simulink library "eng_simple_transient_std"  (Simulink 8.7)
settings: Solver=ode45  StartTime=0.0  StopTime=10.0  RelTol=1e-3
undefined symbols (not defined in the file): DiscIntNeverNeededParam, sMP
libraries: simulink x17
(part 1 of 3)
settings Model: Creator=rafrey5  LastModifiedBy=gerhajo

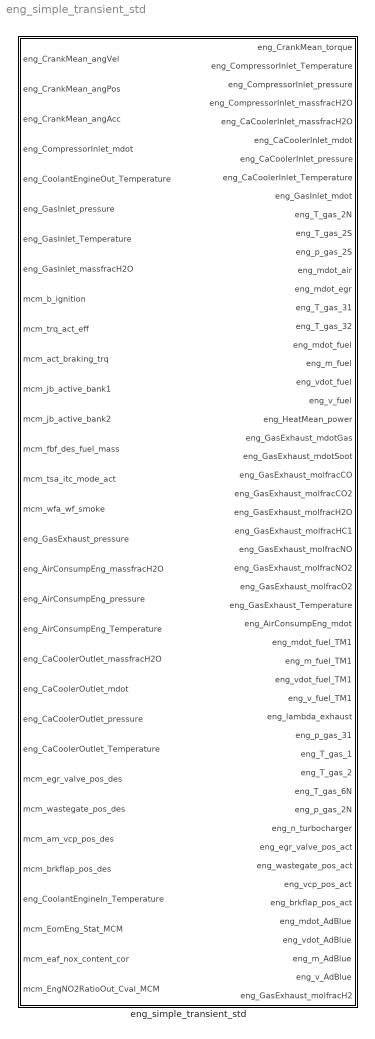
== system eng_simple_transient_std ==
  eng_simple_transient_std : Subsystem  TreatAsAtomicUnit=on  SystemSampleTime=0.01  mask{Airpath_EGRcooler_x_EGR_flow=sMP.phys.eng.Airpath_EGRcooler_x_EGR_flow, Airpath_EGRcooler_y_delta_Temp=sMP.phys.eng.Airpath_EGRcooler_y_delta_Temp, Airpath_EGRcooler_z_efficiency=sMP.phys.eng.Airpath_EGRcooler_z_efficiency, Airpath_Pdrop_aftTurb_coeff=sMP.phys.eng.Airpath_Pdrop_aftTurb_coeff, Airpath_Pdrop_aircooler_coeff=sMP.phys.eng.Airpath_Pdrop_aircooler_coeff, Airpath_Pdrop_aircooler_coeffBr_a1=sMP.phys.eng.Airpath_Pdrop_aircooler_coeffBr_a1, Airpath_Pdrop_aircooler_coeffBr_a2=sMP.phys.eng.Airpath_Pdrop_aircooler_coeffBr_a2, Airpath_Pdrop_bfrComp_coeff=sMP.phys.eng.Airpath_Pdrop_bfrComp_coeff, Airpath_Tairbox_EGR_coeff=sMP.phys.eng.Airpath_Tairbox_EGR_coeff, Airpath_aircooler_x_ML_kgh=sMP.phys.eng.Airpath_aircooler_x_ML_kgh, Airpath_aircooler_y_delta_Temp=sMP.phys.eng.Airpath_aircooler_y_delta_Temp, Airpath_aircooler_z_efficiency=sMP.phys.eng.Airpath_aircooler_z_efficiency, Airpath_compressor_x_massFlow_kgh=sMP.phys.eng.Airpath_compressor_x_massFlow_kgh, Airpath_compressor_y_PressRatio=sMP.phys.eng.Airpath_compressor_y_PressRatio, Airpath_compressor_z_Efficiency=sMP.phys.eng.Airpath_compressor_z_Efficiency, Airpath_intakeflow_x_NMOTW_rpm=sMP.phys.eng.Airpath_intakeflow_x_NMOTW_rpm, Airpath_intakeflow_y_P2S_mbar=sMP.phys.eng.Airpath_intakeflow_y_P2S_mbar, Airpath_intakeflow_z_VolEff=sMP.phys.eng.Airpath_intakeflow_z_VolEff, Airpath_turbine_x_PressRatio=sMP.phys.eng.Airpath_turbine_x_PressRatio, Airpath_turbine_y_Efficiency=sMP.phys.eng.Airpath_turbine_y_Efficiency, ECU_torque_x_NMOT_rpm=sMP.phys.eng.ECU_torque_x_NMOT_rpm, ECU_torque_y_FrictionLine_MISTEE_Nm=sMP.phys.eng.ECU_torque_y_FrictionLine_MISTEE_Nm, ECU_torque_y_FullLoad_MISTEE_Nm=sMP.phys.eng.ECU_torque_y_FullLoad_MISTEE_Nm, Eng_characteristics_AdBlue_density=sMP.phys.eng.Eng_characteristics_AdBlue_density, Eng_characteristics_Fuel_density=sMP.phys.eng.Eng_characteristics_Fuel_density, Eng_characteristics_Mfuel_available=sMP.phys.eng.Eng_characteristics_Mfuel_available, Eng_characteristics_Mfuel_with_MCM=sMP.phys.eng.Eng_characteristics_Mfuel_with_MCM, Eng_characteristics_Stoech_coeff=sMP.phys.eng.Eng_characteristics_Stoech_coeff, Eng_characteristics_V_cylinder=sMP.phys.eng.Eng_characteristics_V_cylinder, Eng_characteristics_assymTurbine=sMP.phys.eng.Eng_characteristics_assymTurbine, Eng_characteristics_n_cylinder=sMP.phys.eng.Eng_characteristics_n_cylinder, Eng_characteristics_use_mcm_NOx=sMP.phys.eng.Eng_characteristics_use_mcm_NOx, Eng_initialisation_eng_started=sMP.phys.eng.Eng_initialisation_eng_started, Eng_starter_fuelInj_minEngSpd=sMP.phys.eng.Eng_starter_fuelInj_minEngSpd, Eng_starter_fuel_penalty_kg=sMP.phys.eng.Eng_starter_fuel_penalty_kg, Eng_starter_time_constant=sMP.phys.eng.Eng_starter_time_constant, Eng_starter_torque_Nm=sMP.phys.eng.Eng_starter_torque_Nm, Fiter_calibration_brmode_x_NMOT_rpm=sMP.phys.eng.Fiter_calibration_brmode_x_NMOT_rpm, Fiter_calibration_brmode_y_tc_P2S=sMP.phys.eng.Fiter_calibration_brmode_y_tc_P2S, Fiter_calibration_brmode_y_tc_P31=sMP.phys.eng.Fiter_calibration_brmode_y_tc_P31, Fiter_calibration_brmode_y_tc_P32=sMP.phys.eng.Fiter_calibration_brmode_y_tc_P32, Fiter_calibration_brmode_y_tc_T31=sMP.phys.eng.Fiter_calibration_brmode_y_tc_T31, Fiter_calibration_brmode_y_tc_T32=sMP.phys.eng.Fiter_calibration_brmode_y_tc_T32, Fiter_calibration_dt=sMP.phys.eng.Fiter_calibration_dt, Fiter_calibration_fmode_x_NMOT_rpm=sMP.phys.eng.Fiter_calibration_fmode_x_NMOT_rpm, Fiter_calibration_fmode_y_ec_EGRTAT=sMP.phys.eng.Fiter_calibration_fmode_y_ec_EGRTAT, Fiter_calibration_fmode_y_tc_EGRTAT=sMP.phys.eng.Fiter_calibration_fmode_y_tc_EGRTAT, Fiter_calibration_fmode_y_tc_P2S_dc=sMP.phys.eng.Fiter_calibration_fmode_y_tc_P2S_dc, Fiter_calibration_fmode_y_tc_P2S_ic=sMP.phys.eng.Fiter_calibration_fmode_y_tc_P2S_ic, Fiter_calibration_fmode_y_tc_P31_dc=sMP.phys.eng.Fiter_calibration_fmode_y_tc_P31_dc, Fiter_calibration_fmode_y_tc_P31_ic=sMP.phys.eng.Fiter_calibration_fmode_y_tc_P31_ic, Fiter_calibration_fmode_y_tc_P32_dc=sMP.phys.eng.Fiter_calibration_fmode_y_tc_P32_dc, Fiter_calibration_fmode_y_tc_P32_ic=sMP.phys.eng.Fiter_calibration_fmode_y_tc_P32_ic, Fiter_calibration_fmode_y_tc_T2N=sMP.phys.eng.Fiter_calibration_fmode_y_tc_T2N, Fiter_calibration_fmode_y_tc_T2V=sMP.phys.eng.Fiter_calibration_fmode_y_tc_T2V, Fiter_calibration_fmode_y_tc_T31_dc=sMP.phys.eng.Fiter_calibration_fmode_y_tc_T31_dc, Fiter_calibration_fmode_y_tc_T31_ic=sMP.phys.eng.Fiter_calibration_fmode_y_tc_T31_ic, Fiter_calibration_fmode_y_tc_T32_dc=sMP.phys.eng.Fiter_calibration_fmode_y_tc_T32_dc, Fiter_calibration_fmode_y_tc_T32_ic=sMP.phys.eng.Fiter_calibration_fmode_y_tc_T32_ic, Setpoint_brakingMode1_x_NMOTW_rpm=sMP.phys.eng.Setpoint_brakingMode1_x_NMOTW_rpm, Setpoint_brakingMode1_y_alphaTorque=sMP.phys.eng.Setpoint_brakingMode1_y_alphaTorque, Setpoint_brakingMode1_z_P2S_mbar=sMP.phys.eng.Setpoint_brakingMode1_z_P2S_mbar, Setpoint_brakingMode1_z_P31_mbar=sMP.phys.eng.Setpoint_brakingMode1_z_P31_mbar, Setpoint_brakingMode1_z_T31_degC=sMP.phys.eng.Setpoint_brakingMode1_z_T31_degC, Setpoint_brakingMode1_z_Torque_Nm=sMP.phys.eng.Setpoint_brakingMode1_z_Torque_Nm, Setpoint_brakingMode2_x_NMOTW_rpm=sMP.phys.eng.Setpoint_brakingMode2_x_NMOTW_rpm, Setpoint_brakingMode2_y_alphaTorque=sMP.phys.eng.Setpoint_brakingMode2_y_alphaTorque, Setpoint_brakingMode2_z_P2S_mbar=sMP.phys.eng.Setpoint_brakingMode2_z_P2S_mbar, Setpoint_brakingMode2_z_P32_mbar=sMP.phys.eng.Setpoint_brakingMode2_z_P32_mbar, Setpoint_brakingMode2_z_T32_degC=sMP.phys.eng.Setpoint_brakingMode2_z_T32_degC, Setpoint_brakingMode2_z_Torque_Nm=sMP.phys.eng.Setpoint_brakingMode2_z_Torque_Nm, Setpoint_brakingMode3_x_NMOTW_rpm=sMP.phys.eng.Setpoint_brakingMode3_x_NMOTW_rpm, Setpoint_brakingMode3_y_alphaTorque=sMP.phys.eng.Setpoint_brakingMode3_y_alphaTorque, Setpoint_brakingMode3_z_EGRTAT=sMP.phys.eng.Setpoint_brakingMode3_z_EGRTAT, Setpoint_brakingMode3_z_P2S_mbar=sMP.phys.eng.Setpoint_brakingMode3_z_P2S_mbar, Setpoint_brakingMode3_z_P31_mbar=sMP.phys.eng.Setpoint_brakingMode3_z_P31_mbar, Setpoint_brakingMode3_z_P32_mbar=sMP.phys.eng.Setpoint_brakingMode3_z_P32_mbar, Setpoint_brakingMode3_z_T31_degC=sMP.phys.eng.Setpoint_brakingMode3_z_T31_degC, Setpoint_brakingMode3_z_T32_degC=sMP.phys.eng.Setpoint_brakingMode3_z_T32_degC, Setpoint_brakingMode3_z_Torque_Nm=sMP.phys.eng.Setpoint_brakingMode3_z_Torque_Nm, Setpoint_fuelledMode_x_NMOTW_rpm=sMP.phys.eng.Setpoint_fuelledMode_x_NMOTW_rpm, Setpoint_fuelledMode_y_alphaTorque=sMP.phys.eng.Setpoint_fuelledMode_y_alphaTorque, Setpoint_fuelledMode_z_CO_ppm=sMP.phys.eng.Setpoint_fuelledMode_z_CO_ppm, Setpoint_fuelledMode_z_dMFueldT2N=sMP.phys.eng.Setpoint_fuelledMode_z_dMFueldT2N, Setpoint_fuelledMode_z_dMFueldTWE=sMP.phys.eng.Setpoint_fuelledMode_z_dMFueldTWE, Setpoint_fuelledMode_z_EGRTAT=sMP.phys.eng.Setpoint_fuelledMode_z_EGRTAT, Setpoint_fuelledMode_z_HC_ppm=sMP.phys.eng.Setpoint_fuelledMode_z_HC_ppm, Setpoint_fuelledMode_z_MAdBlue_kgh=sMP.phys.eng.Setpoint_fuelledMode_z_MAdBlue_kgh, Setpoint_fuelledMode_z_Mfuel_mgstr=sMP.phys.eng.Setpoint_fuelledMode_z_Mfuel_mgstr, Setpoint_fuelledMode_z_Mfuel_TM1_mgstr=sMP.phys.eng.Setpoint_fuelledMode_z_Mfuel_TM1_mgstr, Setpoint_fuelledMode_z_Mfuel_smoke_factor=sMP.phys.eng.Setpoint_fuelledMode_z_Mfuel_smoke_factor, Setpoint_fuelledMode_z_NO_ppm=sMP.phys.eng.Setpoint_fuelledMode_z_NO_ppm, Setpoint_fuelledMode_z_NOx_ppm=sMP.phys.eng.Setpoint_fuelledMode_z_NOx_ppm, Setpoint_fuelledMode_z_P2S_mbar=sMP.phys.eng.Setpoint_fuelledMode_z_P2S_mbar, Setpoint_fuelledMode_z_P31_mbar=sMP.phys.eng.Setpoint_fuelledMode_z_P31_mbar, Setpoint_fuelledMode_z_P32_mbar=sMP.phys.eng.Setpoint_fuelledMode_z_P32_mbar, Setpoint_fuelledMode_z_T2N_degC=sMP.phys.eng.Setpoint_fuelledMode_z_T2N_degC, Setpoint_fuelledMode_z_T31_degC=sMP.phys.eng.Setpoint_fuelledMode_z_T31_degC, Setpoint_fuelledMode_z_T32_degC=sMP.phys.eng.Setpoint_fuelledMode_z_T32_degC, Setpoint_fuelledMode_z_TWE_degC=sMP.phys.eng.Setpoint_fuelledMode_z_TWE_degC, Setpoint_fuelledMode_z_Torque_Nm=sMP.phys.eng.Setpoint_fuelledMode_z_Torque_Nm, Thermal_heatRelease_negTorque_factor=sMP.phys.eng.Thermal_heatRelease_negTorque_factor, Thermal_heatRelease_x_NMOT_rpm=sMP.phys.eng.Thermal_heatRelease_x_NMOT_rpm, Thermal_heatRelease_y_Torque_Nm=sMP.phys.eng.Thermal_heatRelease_y_Torque_Nm, Thermal_heatRelease_z_heat_kW=sMP.phys.eng.Thermal_heatRelease_z_heat_kW, egr_smoke_lim_x_NMOT_rpm=sMP.phys.eng.egr_smoke_lim_x_NMOT_rpm, egr_smoke_lim_y_Mfuel_mgstr=sMP.phys.eng.egr_smoke_lim_y_Mfuel_mgstr, egr_smoke_lim_z_desAir_kgh=sMP.phys.eng.egr_smoke_lim_z_desAir_kgh, egr_smoke_lim_z_minAFR=sMP.phys.eng.egr_smoke_lim_z_minAFR, tc_speed_calc_3m=sMP.phys.eng.tc_speed_calc_3m, tc_speed_calc_x_p_intake=sMP.phys.eng.tc_speed_calc_x_p_intake, tc_speed_calc_y_eng_speed=sMP.phys.eng.tc_speed_calc_y_eng_speed}
      mask init:
      | 0.01;
      mask Display: disp(['Fast engine model' char(10) 'Release date :' char(10) '2021 / 07 / 21'])

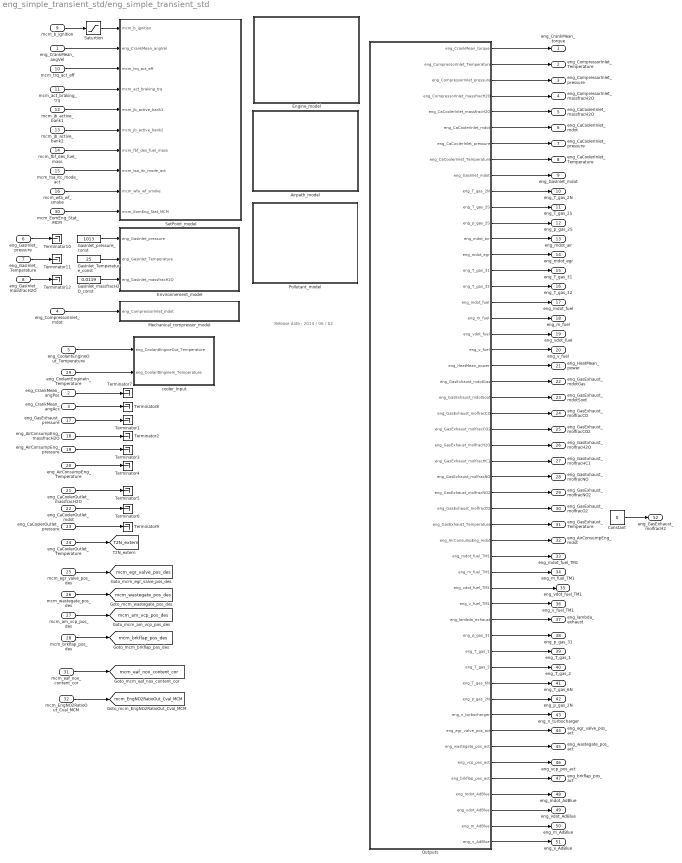
== system eng_simple_transient_std/eng_simple_transient_std ==
  note: Release date :
      | 2014 / 06 / 02
  eng_CrankMean_angVel : Inport
  eng_CrankMean_angPos : Inport  Port=2
  eng_CrankMean_angAcc : Inport  Port=3
  eng_CompressorInlet_mdot : Inport  Port=4
  eng_CoolantEngineOut_Temperature : Inport  Port=5
  eng_GasInlet_pressure : Inport  Port=6
  eng_GasInlet_Temperature : Inport  Port=7
  eng_GasInlet_massfracH2O : Inport  Port=8
  mcm_b_ignition : Inport  Port=9
  mcm_trq_act_eff : Inport  Port=10
  mcm_act_braking_trq : Inport  Port=11
  mcm_jb_active_bank1 : Inport  Port=12
  mcm_jb_active_bank2 : Inport  Port=13
  mcm_fbf_des_fuel_mass : Inport  Port=14
  mcm_tsa_itc_mode_act : Inport  Port=15
  mcm_wfa_wf_smoke : Inport  Port=16
  eng_GasExhaust_pressure : Inport  Port=17
  eng_AirConsumpEng_massfracH2O : Inport  Port=18
  eng_AirConsumpEng_pressure : Inport  Port=19
  eng_AirConsumpEng_Temperature : Inport  Port=20
  eng_CaCoolerOutlet_massfracH2O : Inport  Port=21
  eng_CaCoolerOutlet_mdot : Inport  Port=22
  eng_CaCoolerOutlet_pressure : Inport  Port=23
  eng_CaCoolerOutlet_Temperature : Inport  Port=24
  mcm_egr_valve_pos_des : Inport  Port=25
  mcm_wastegate_pos_des : Inport  Port=26
  mcm_am_vcp_pos_des : Inport  Port=27
  mcm_brkflap_pos_des : Inport  Port=28
  eng_CoolantEngineIn_Temperature : Inport  Port=29
  mcm_EomEng_Stat_MCM : Inport  Port=30
  mcm_eaf_nox_content_cor : Inport  Port=31
  mcm_EngNO2RatioOut_Cval_MCM : Inport  Port=32
  Airpath_model : Subsystem
  Constant : Constant  Value=0
  Engine_model : Subsystem
  Environnement_model : Subsystem
  GasInlet_Temperature_const : Constant  Value=25
  GasInlet_massfracH2O_const : Constant  Value=0.0119
  GasInlet_pressure_const : Constant  Value=1013
  Mechanical_compressor_model : Subsystem
  Outputs : Subsystem
  Pollutant_model : Subsystem
  Saturtion : Saturate  UpperLimit=1  LowerLimit=1
  SetPoint_model : Subsystem
  Terminator{1..12} (12 alike) : Terminator
  cooler_Input : Subsystem
  eng_CrankMean_torque : Outport
  eng_CompressorInlet_Temperature : Outport  Port=2
  eng_CompressorInlet_pressure : Outport  Port=3
  eng_CompressorInlet_massfracH2O : Outport  Port=4
  eng_CaCoolerInlet_massfracH2O : Outport  Port=5
  eng_CaCoolerInlet_mdot : Outport  Port=6
  eng_CaCoolerInlet_pressure : Outport  Port=7
  eng_CaCoolerInlet_Temperature : Outport  Port=8
  eng_GasInlet_mdot : Outport  Port=9
  eng_T_gas_2N : Outport  Port=10
  eng_T_gas_2S : Outport  Port=11
  eng_p_gas_2S : Outport  Port=12
  eng_mdot_air : Outport  Port=13
  eng_mdot_egr : Outport  Port=14
  eng_T_gas_31 : Outport  Port=15
  eng_T_gas_32 : Outport  Port=16
  eng_mdot_fuel : Outport  Port=17
  eng_m_fuel : Outport  Port=18
  eng_vdot_fuel : Outport  Port=19
  eng_v_fuel : Outport  Port=20
  eng_HeatMean_power : Outport  Port=21
  eng_GasExhaust_mdotGas : Outport  Port=22
  eng_GasExhaust_mdotSoot : Outport  Port=23
  eng_GasExhaust_molfracCO : Outport  Port=24
  eng_GasExhaust_molfracCO2 : Outport  Port=25
  eng_GasExhaust_molfracH2O : Outport  Port=26
  eng_GasExhaust_molfracHC1 : Outport  Port=27
  eng_GasExhaust_molfracNO : Outport  Port=28
  eng_GasExhaust_molfracNO2 : Outport  Port=29
  eng_GasExhaust_molfracO2 : Outport  Port=30
  eng_GasExhaust_Temperature : Outport  Port=31
  eng_AirConsumpEng_mdot : Outport  Port=32
  eng_mdot_fuel_TM1 : Outport  Port=33
  eng_m_fuel_TM1 : Outport  Port=34
  eng_vdot_fuel_TM1 : Outport  Port=35
  eng_v_fuel_TM1 : Outport  Port=36
  eng_lambda_exhaust : Outport  Port=37
  eng_p_gas_31 : Outport  Port=38
  eng_T_gas_1 : Outport  Port=39
  eng_T_gas_2 : Outport  Port=40
  eng_T_gas_6N : Outport  Port=41
  eng_p_gas_2N : Outport  Port=42
  eng_n_turbocharger : Outport  Port=43
  eng_egr_valve_pos_act : Outport  Port=44
  eng_wastegate_pos_act : Outport  Port=45
  eng_vcp_pos_act : Outport  Port=46
  eng_brkflap_pos_act : Outport  Port=47
  eng_mdot_AdBlue : Outport  Port=48
  eng_vdot_AdBlue : Outport  Port=49
  eng_m_AdBlue : Outport  Port=50
  eng_v_AdBlue : Outport  Port=51
  eng_GasExhaust_molfracH2 : Outport  Port=52
  tag scope: T2N_extern=global, mcm_EngNO2RatioOut_Cval_MCM=global, mcm_am_vcp_pos_des=global, mcm_brkflap_pos_des=global, mcm_eaf_nox_content_cor=global, mcm_egr_valve_pos_des=global, mcm_wastegate_pos_des=global
  wires:
  eng_CompressorInlet_mdot/1 -> Mechanical_compressor_model/1(eng_CompressorInlet_mdot)
  eng_CrankMean_angVel/1 -> SetPoint_model/2(eng_CrankMean_angVel)
  eng_CrankMean_angAcc/1 -> Terminator8/1
  eng_CrankMean_angPos/1 -> Terminator7/1
  eng_CoolantEngineOut_Temperature/1 -> cooler_Input/1(eng_CoolantEngineOut_Temperature)
  mcm_fbf_des_fuel_mass/1 -> SetPoint_model/7(mcm_fbf_des_fuel_mass)
  mcm_jb_active_bank2/1 -> SetPoint_model/6(mcm_jb_active_bank2)
  mcm_jb_active_bank1/1 -> SetPoint_model/5(mcm_jb_active_bank1)
  mcm_act_braking_trq/1 -> SetPoint_model/4(mcm_act_braking_trq)
  mcm_trq_act_eff/1 -> SetPoint_model/3(mcm_trq_act_eff)
  mcm_b_ignition/1 -> Saturtion/1
  eng_GasExhaust_pressure/1 -> Terminator1/1
  eng_AirConsumpEng_massfracH2O/1 -> Terminator2/1
  eng_AirConsumpEng_pressure/1 -> Terminator3/1
  eng_AirConsumpEng_Temperature/1 -> Terminator4/1
  Saturtion/1 -> SetPoint_model/1(mcm_b_ignition)
  mcm_tsa_itc_mode_act/1 -> SetPoint_model/8(mcm_tsa_itc_mode_act)
  mcm_wfa_wf_smoke/1 -> SetPoint_model/9(mcm_wfa_wf_smoke)
  Outputs/1(eng_CrankMean_torque) -> eng_CrankMean_torque/1
  Outputs/2(eng_CompressorInlet_Temperature) -> eng_CompressorInlet_Temperature/1
  Outputs/3(eng_CompressorInlet_pressure) -> eng_CompressorInlet_pressure/1
  Outputs/4(eng_CompressorInlet_massfracH2O) -> eng_CompressorInlet_massfracH2O/1
  Outputs/5(eng_CaCoolerInlet_massfracH2O) -> eng_CaCoolerInlet_massfracH2O/1
  Outputs/6(eng_CaCoolerInlet_mdot) -> eng_CaCoolerInlet_mdot/1
  Outputs/7(eng_CaCoolerInlet_pressure) -> eng_CaCoolerInlet_pressure/1
  Outputs/8(eng_CaCoolerInlet_Temperature) -> eng_CaCoolerInlet_Temperature/1
  Outputs/9(eng_GasInlet_mdot) -> eng_GasInlet_mdot/1
  Outputs/10(eng_T_gas_2N) -> eng_T_gas_2N/1
  Outputs/11(eng_T_gas_2S) -> eng_T_gas_2S/1
  Outputs/12(eng_p_gas_2S) -> eng_p_gas_2S/1
  Outputs/13(eng_mdot_air) -> eng_mdot_air/1
  Outputs/14(eng_mdot_egr) -> eng_mdot_egr/1
  Outputs/15(eng_T_gas_31) -> eng_T_gas_31/1
  Outputs/16(eng_T_gas_32) -> eng_T_gas_32/1
  Outputs/17(eng_mdot_fuel) -> eng_mdot_fuel/1
  Outputs/18(eng_m_fuel) -> eng_m_fuel/1
  Outputs/19(eng_vdot_fuel) -> eng_vdot_fuel/1
  Outputs/20(eng_v_fuel) -> eng_v_fuel/1
  Outputs/21(eng_HeatMean_power) -> eng_HeatMean_power/1
  Outputs/22(eng_GasExhaust_mdotGas) -> eng_GasExhaust_mdotGas/1
  Outputs/23(eng_GasExhaust_mdotSoot) -> eng_GasExhaust_mdotSoot/1
  Outputs/24(eng_GasExhaust_molfracCO) -> eng_GasExhaust_molfracCO/1
  Outputs/25(eng_GasExhaust_molfracCO2) -> eng_GasExhaust_molfracCO2/1
  Outputs/26(eng_GasExhaust_molfracH2O) -> eng_GasExhaust_molfracH2O/1
  Outputs/27(eng_GasExhaust_molfracHC1) -> eng_GasExhaust_molfracHC1/1
  Outputs/28(eng_GasExhaust_molfracNO) -> eng_GasExhaust_molfracNO/1
  Outputs/29(eng_GasExhaust_molfracNO2) -> eng_GasExhaust_molfracNO2/1
  Outputs/30(eng_GasExhaust_molfracO2) -> eng_GasExhaust_molfracO2/1
  Outputs/31(eng_GasExhaust_Temperature) -> eng_GasExhaust_Temperature/1
  Outputs/32(eng_AirConsumpEng_mdot) -> eng_AirConsumpEng_mdot/1
  eng_CaCoolerOutlet_massfracH2O/1 -> Terminator5/1
  eng_CaCoolerOutlet_mdot/1 -> Terminator6/1
  eng_CaCoolerOutlet_pressure/1 -> Terminator9/1
  eng_CaCoolerOutlet_Temperature/1 -> [T2N_extern]
  Outputs/33(eng_mdot_fuel_TM1) -> eng_mdot_fuel_TM1/1
  Outputs/34(eng_m_fuel_TM1) -> eng_m_fuel_TM1/1
  Outputs/35(eng_vdot_fuel_TM1) -> eng_vdot_fuel_TM1/1
  Outputs/36(eng_v_fuel_TM1) -> eng_v_fuel_TM1/1
  Outputs/37(eng_lambda_exhaust) -> eng_lambda_exhaust/1
  Outputs/38(eng_p_gas_31) -> eng_p_gas_31/1
  Outputs/39(eng_T_gas_1) -> eng_T_gas_1/1
  Outputs/40(eng_T_gas_2) -> eng_T_gas_2/1
  Outputs/41(eng_T_gas_6N) -> eng_T_gas_6N/1
  Outputs/42(eng_p_gas_2N) -> eng_p_gas_2N/1
  Outputs/43(eng_n_turbocharger) -> eng_n_turbocharger/1
  mcm_egr_valve_pos_des/1 -> [mcm_egr_valve_pos_des]
  mcm_wastegate_pos_des/1 -> [mcm_wastegate_pos_des]
  mcm_am_vcp_pos_des/1 -> [mcm_am_vcp_pos_des]
  mcm_brkflap_pos_des/1 -> [mcm_brkflap_pos_des]
  Outputs/44(eng_egr_valve_pos_act) -> eng_egr_valve_pos_act/1
  Outputs/45(eng_wastegate_pos_act) -> eng_wastegate_pos_act/1
  Outputs/46(eng_vcp_pos_act) -> eng_vcp_pos_act/1
  Outputs/47(eng_brkflap_pos_act) -> eng_brkflap_pos_act/1
  Outputs/48(eng_mdot_AdBlue) -> eng_mdot_AdBlue/1
  Outputs/49(eng_vdot_AdBlue) -> eng_vdot_AdBlue/1
  Outputs/50(eng_m_AdBlue) -> eng_m_AdBlue/1
  Outputs/51(eng_v_AdBlue) -> eng_v_AdBlue/1
  eng_CoolantEngineIn_Temperature/1 -> cooler_Input/2(eng_CoolantEngineIn_Temperature)
  mcm_EomEng_Stat_MCM/1 -> SetPoint_model/10(mcm_EomEng_Stat_MCM)
  mcm_eaf_nox_content_cor/1 -> [mcm_eaf_nox_content_cor]
  mcm_EngNO2RatioOut_Cval_MCM/1 -> [mcm_EngNO2RatioOut_Cval_MCM]
  Constant/1 -> eng_GasExhaust_molfracH2/1
  eng_GasInlet_massfracH2O/1 -> Terminator12/1
  eng_GasInlet_Temperature/1 -> Terminator11/1
  eng_GasInlet_pressure/1 -> Terminator10/1
  GasInlet_Temperature_const/1 -> Environnement_model/2(eng_GasInlet_Temperature)
  GasInlet_pressure_const/1 -> Environnement_model/1(eng_GasInlet_pressure)
  GasInlet_massfracH2O_const/1 -> Environnement_model/3(eng_GasInlet_massfracH2O)

== system eng_simple_transient_std/eng_simple_transient_std/Airpath_model ==
  After EGR cooler calculation : Subsystem
  After air cooler calculation : Subsystem
  After compressor calculation : Subsystem
  After turbine calculation : Subsystem
  Airbox calculation : Subsystem
  Before EGR cooler calculation : Subsystem
  Before compressor calculation : Subsystem
  Before turbine calculation : Subsystem
  Bus Creator4 : BusCreator  Inputs=22
  Intake flows calculation : Subsystem
  tag scope: Airpath=global
  wires:
  Before turbine calculation/4(T32_degC) -> Bus Creator4/16  "T32_degC"
  Before turbine calculation/3(P32_mbar) -> Bus Creator4/15  "P32_mbar"
  After EGR cooler calculation/2(T6N_degC) -> Bus Creator4/22  "T6N_degC"
  After EGR cooler calculation/1(P6N_mbar) -> Bus Creator4/21  "P6N_mbar"
  Before EGR cooler calculation/2(T6V_degC) -> Bus Creator4/20  "T6V_degC"
  Before EGR cooler calculation/1(P6V_mbar) -> Bus Creator4/19  "P6V_mbar"
  After turbine calculation/2(T4_degC) -> Bus Creator4/18  "T4_degC"
  After turbine calculation/1(P4_mbar) -> Bus Creator4/17  "P4_mbar"
  Before turbine calculation/2(T31_degC) -> Bus Creator4/14  "T31_degC"
  Before turbine calculation/1(P31_mbar) -> Bus Creator4/13  "P31_mbar"
  Airbox calculation/2(T2S_degC) -> Bus Creator4/12  "T2S_degC"
  Airbox calculation/1(P2S_mbar) -> Bus Creator4/11  "P2S_mbar"
  After air cooler calculation/2(T2N_degC) -> Bus Creator4/10  "T2N_degC"
  After air cooler calculation/1(P2N_mbar) -> Bus Creator4/9  "P2N_mbar"
  After compressor calculation/2(T2V_degC) -> Bus Creator4/8  "T2V_degC"
  After compressor calculation/1(P2V_mbar) -> Bus Creator4/7  "P2V_mbar"
  Before compressor calculation/3(T1_degC) -> Bus Creator4/6  "T1_degC"
  Before compressor calculation/2(P1_mbar) -> Bus Creator4/5  "P1_mbar"
  Before compressor calculation/1(massfracH2O) -> Bus Creator4/4  "massfracH2O"
  Intake flows calculation/3(EGRTAT) -> Bus Creator4/3  "EGRTAT"
  Intake flows calculation/2(EGR_flow_kgh) -> Bus Creator4/2  "EGRflow_kgh"
  Intake flows calculation/1(Air_mass_flow_kgh) -> Bus Creator4/1  "AirMassFlow_kgh"
  Bus Creator4/1 -> [Airpath]  "Airpath"

== system eng_simple_transient_std/eng_simple_transient_std/Engine_model ==
  AFR calculation : Subsystem
  AdBlue consumption : Subsystem
  Bus Creator4 : BusCreator  Inputs=17
  Fuel consumption calculation : Subsystem
  cooler_model : Subsystem
  tag scope: Engine=global
  wires:
  Bus Creator4/1 -> [Engine]  "Engine"
  Fuel consumption calculation/2(VFuel_Lh) -> Bus Creator4/4  "Vfuel_Lh"
  Fuel consumption calculation/4(VFuel_L) -> Bus Creator4/6  "Vfuel_L"
  Fuel consumption calculation/3(MFuel_kg) -> Bus Creator4/5  "Mfuel_kg"
  Fuel consumption calculation/1(MFuel_kgh) -> Bus Creator4/3  "Mfuel_kgh"
  [Mfuel_mgstr] -> Bus Creator4/2  "Mfuel_mgstr"
  [Torque_Nm_sp] -> Bus Creator4/1  "Torque_Nm"
  Fuel consumption calculation/5(MFuel_TM1_kgh) -> Bus Creator4/7  "Mfuel_TM1_kgh"
  Fuel consumption calculation/6(VFuel_TM1_Lh) -> Bus Creator4/8  "Vfuel_TM1_Lh"
  Fuel consumption calculation/7(MFuel_TM1_kg) -> Bus Creator4/9  "Mfuel_TM1_kg"
  Fuel consumption calculation/8(VFuel_TM1_L) -> Bus Creator4/10  "Vfuel_TM1_L"
  AFR calculation/1(AFR) -> Bus Creator4/11  "AFR"
  cooler_model/1(eng_HeatMean_power) -> Bus Creator4/12
  [EngSpeed] -> Bus Creator4/13  "EngSpeed_rpm"
  AdBlue consumption/1(MAdBlue_brk_kgh) -> Bus Creator4/14  "MAdBlue_kgh"
  AdBlue consumption/2(VAdBlue_Lh) -> Bus Creator4/15  "VAdBlue_Lh"
  AdBlue consumption/3(MAdBlue_kg) -> Bus Creator4/16  "MAdBlue_kg"
  AdBlue consumption/4(VAdBlue_L) -> Bus Creator4/17  "VAdBlue_L"

== system eng_simple_transient_std/eng_simple_transient_std/Environnement_model ==
  eng_GasInlet_pressure : Inport
  eng_GasInlet_Temperature : Inport  Port=2
  eng_GasInlet_massfracH2O : Inport  Port=3
  tag scope: env_AirH2OMassFrac=global, env_AirPress=global, env_AirTemp=global
  wires:
  eng_GasInlet_massfracH2O/1 -> [env_AirH2OMassFrac]
  eng_GasInlet_Temperature/1 -> [env_AirTemp]
  eng_GasInlet_pressure/1 -> [env_AirPress]

== system eng_simple_transient_std/eng_simple_transient_std/Mechanical_compressor_model ==
  eng_CompressorInlet_mdot : Inport
  Terminator : Terminator
  wires:
  eng_CompressorInlet_mdot/1 -> Terminator/1

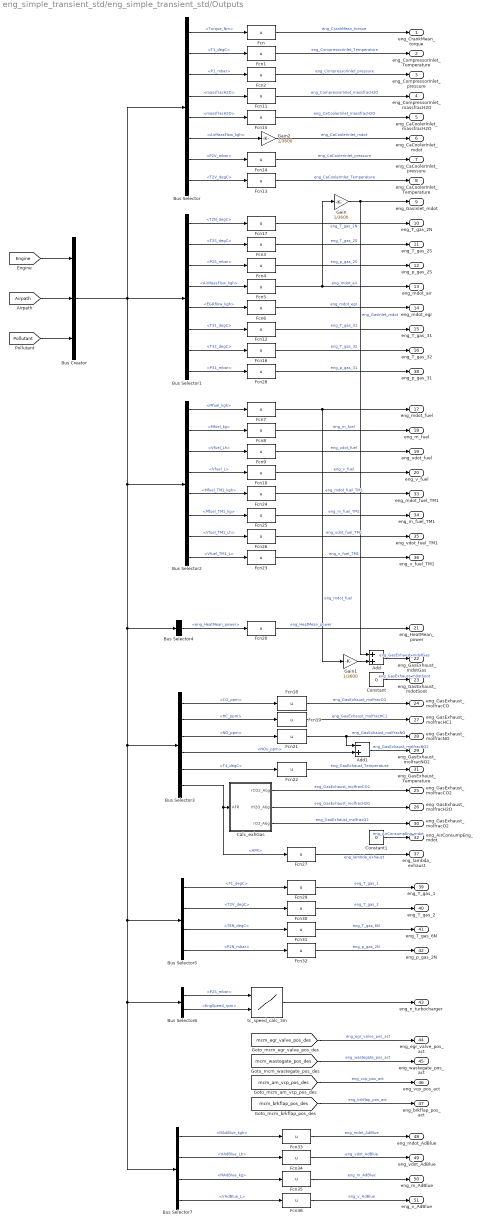
== system eng_simple_transient_std/eng_simple_transient_std/Outputs ==
  Add : Sum
  Add1 : Sum  Inputs=-+
  Bus Creator : BusCreator  Inputs=3
  Bus Selector : BusSelector  OutputSignals=Engine.Torque_Nm,Airpath.T1_degC,Airpath.P1_mbar,Airpath.massfracH2O,Airpath.massfracH2O,Airpath.AirMassFlow_kgh,Airpath.P2V_mbar,Airpath.T2V_degC
  Bus Selector1 : BusSelector  OutputSignals=Airpath.T2N_degC,Airpath.T2S_degC,Airpath.P2S_mbar,Airpath.AirMassFlow_kgh,Airpath.EGRflow_kgh,Airpath.T31_degC,Airpath.T32_degC,Airpath.P31_mbar
  Bus Selector2 : BusSelector  OutputSignals=Engine.Mfuel_kgh,Engine.Mfuel_kg,Engine.Vfuel_Lh,Engine.Vfuel_L,Engine.Mfuel_TM1_kgh,Engine.Mfuel_TM1_kg,Engine.Vfuel_TM1_Lh,Engine.Vfuel_TM1_L
  Bus Selector3 : BusSelector  OutputSignals=Pollutant.CO_ppm,Pollutant.HC_ppm,Pollutant.NO_ppm,Pollutant.NOx_ppm,Airpath.T4_degC,Engine.AFR
  Bus Selector4 : BusSelector  OutputSignals=Engine.eng_HeatMean_power
  Bus Selector5 : BusSelector  OutputSignals=Airpath.T1_degC,Airpath.T2V_degC,Airpath.T6N_degC,Airpath.P2N_mbar
  Bus Selector6 : BusSelector  OutputSignals=Airpath.P2S_mbar,Engine.EngSpeed_rpm
  Bus Selector7 : BusSelector  OutputSignals=Engine.MAdBlue_kgh,Engine.VAdBlue_Lh,Engine.MAdBlue_kg,Engine.VAdBlue_L
  Calc_exhGas : Subsystem
  Constant : Constant  Value=0
  Constant1 : Constant  Value=0
  Fcn{,1..36} (37 alike) : Fcn  Expr=u
  Gain : Gain  Gain=1/3600
  Gain1 : Gain  Gain=1/3600
  Gain2 : Gain  Gain=1/3600
  tc_speed_calc_3m : Lookup2D  RowIndex=tc_speed_calc_x_p_intake  ColumnIndex=tc_speed_calc_y_eng_speed  Table=tc_speed_calc_3m  LookUpMeth=Interpolation-Use End Values
  eng_CrankMean_torque : Outport
  eng_CompressorInlet_Temperature : Outport  Port=2
  eng_CompressorInlet_pressure : Outport  Port=3
  eng_CompressorInlet_massfracH2O : Outport  Port=4
  eng_CaCoolerInlet_massfracH2O : Outport  Port=5
  eng_CaCoolerInlet_mdot : Outport  Port=6
  eng_CaCoolerInlet_pressure : Outport  Port=7
  eng_CaCoolerInlet_Temperature : Outport  Port=8
  eng_GasInlet_mdot : Outport  Port=9
  eng_T_gas_2N : Outport  Port=10
  eng_T_gas_2S : Outport  Port=11
  eng_p_gas_2S : Outport  Port=12
  eng_mdot_air : Outport  Port=13
  eng_mdot_egr : Outport  Port=14
  eng_T_gas_31 : Outport  Port=15
  eng_T_gas_32 : Outport  Port=16
  eng_mdot_fuel : Outport  Port=17
  eng_m_fuel : Outport  Port=18
  eng_vdot_fuel : Outport  Port=19
  eng_v_fuel : Outport  Port=20
  eng_HeatMean_power : Outport  Port=21
  eng_GasExhaust_mdotGas : Outport  Port=22
  eng_GasExhaust_mdotSoot : Outport  Port=23
  eng_GasExhaust_molfracCO : Outport  Port=24
  eng_GasExhaust_molfracCO2 : Outport  Port=25
  eng_GasExhaust_molfracH2O : Outport  Port=26
  eng_GasExhaust_molfracHC1 : Outport  Port=27
  eng_GasExhaust_molfracNO : Outport  Port=28
  eng_GasExhaust_molfracNO2 : Outport  Port=29
  eng_GasExhaust_molfracO2 : Outport  Port=30
  eng_GasExhaust_Temperature : Outport  Port=31
  eng_AirConsumpEng_mdot : Outport  Port=32
  eng_mdot_fuel_TM1 : Outport  Port=33
  eng_m_fuel_TM1 : Outport  Port=34
  eng_vdot_fuel_TM1 : Outport  Port=35
  eng_v_fuel_TM1 : Outport  Port=36
  eng_lambda_exhaust : Outport  Port=37
  eng_p_gas_31 : Outport  Port=38
  eng_T_gas_1 : Outport  Port=39
  eng_T_gas_2 : Outport  Port=40
  eng_T_gas_6N : Outport  Port=41
  eng_p_gas_2N : Outport  Port=42
  eng_n_turbocharger : Outport  Port=43
  eng_egr_valve_pos_act : Outport  Port=44
  eng_wastegate_pos_act : Outport  Port=45
  eng_vcp_pos_act : Outport  Port=46
  eng_brkflap_pos_act : Outport  Port=47
  eng_mdot_AdBlue : Outport  Port=48
  eng_vdot_AdBlue : Outport  Port=49
  eng_m_AdBlue : Outport  Port=50
  eng_v_AdBlue : Outport  Port=51
  wires:
  Fcn20/1 -> eng_HeatMean_power/1  "eng_HeatMean_power"
  Fcn10/1 -> eng_v_fuel/1  "eng_v_fuel"
  Fcn9/1 -> eng_vdot_fuel/1  "eng_vdot_fuel"
  Fcn8/1 -> eng_m_fuel/1  "eng_m_fuel"
  Fcn7/1 -> Gain1/1, eng_mdot_fuel/1  "eng_mdot_fuel"
  Fcn6/1 -> eng_mdot_egr/1  "eng_mdot_egr"
  Fcn4/1 -> eng_p_gas_2S/1  "eng_p_gas_2S"
  Fcn3/1 -> eng_T_gas_2S/1  "eng_T_gas_2S"
  Gain/1 -> Add/1, eng_GasInlet_mdot/1  "eng_GasInlet_mdot"
  Bus Selector4/1 -> Fcn20/1  "<eng_HeatMean_power>"
  Bus Selector/4 -> Fcn11/1  "<massfracH2O>"
  Bus Creator/1 -> Bus Selector/1, Bus Selector1/1, Bus Selector2/1, Bus Selector4/1, Bus Selector3/1, Bus Selector5/1, Bus Selector6/1, Bus Selector7/1
  [Pollutant] -> Bus Creator/3
  [Airpath] -> Bus Creator/2
  [Engine] -> Bus Creator/1
  Bus Selector2/4 -> Fcn10/1  "<Vfuel_L>"
  Bus Selector2/3 -> Fcn9/1  "<Vfuel_Lh>"
  Bus Selector2/2 -> Fcn8/1  "<Mfuel_kg>"
  Bus Selector2/1 -> Fcn7/1  "<Mfuel_kgh>"
  Fcn5/1 -> Gain/1, eng_mdot_air/1  "eng_mdot_air"
  Fcn11/1 -> eng_CompressorInlet_massfracH2O/1  "eng_CompressorInlet_massfracH2O"
  Fcn2/1 -> eng_CompressorInlet_pressure/1  "eng_CompressorInlet_pressure"
  Fcn1/1 -> eng_CompressorInlet_Temperature/1  "eng_CompressorInlet_Temperature"
  Fcn/1 -> eng_CrankMean_torque/1  "eng_CrankMean_torque"
  Bus Selector/3 -> Fcn2/1  "<P1_mbar>"
  Bus Selector/2 -> Fcn1/1  "<T1_degC>"
  Bus Selector/1 -> Fcn/1  "<Torque_Nm>"
  Add/1 -> eng_GasExhaust_mdotGas/1  "eng_GasExhaust_mdotGas"
  Gain1/1 -> Add/2
  Constant/1 -> eng_GasExhaust_mdotSoot/1  "eng_GasExhaust_mdotSoot"
  Bus Selector3/1 -> Fcn18/1  "<CO_ppm>"
  Bus Selector3/2 -> Fcn19/1  "<HC_ppm>"
  Bus Selector3/3 -> Fcn21/1  "<NO_ppm>"
  Bus Selector3/4 -> Add1/2  "<NOx_ppm>"
  Bus Selector3/5 -> Fcn22/1  "<T4_degC>"
  Add1/1 -> eng_GasExhaust_molfracNO2/1  "eng_GasExhaust_molfracNO2"
  Bus Selector3/6 -> Calc_exhGas/1(AFR), Fcn27/1  "<AFR>"
  Calc_exhGas/1(rCO2_Abg) -> eng_GasExhaust_molfracCO2/1  "eng_GasExhaust_molfracCO2"
  Calc_exhGas/2(rH2O_Abg) -> eng_GasExhaust_molfracH2O/1  "eng_GasExhaust_molfracH2O"
  Calc_exhGas/3(rO2_Abg) -> eng_GasExhaust_molfracO2/1  "eng_GasExhaust_molfracO2"
  Constant1/1 -> eng_AirConsumpEng_mdot/1  "eng_AirConsumpEng_mdot"
  Bus Selector/8 -> Fcn13/1  "<T2V_degC>"
  Fcn13/1 -> eng_CaCoolerInlet_Temperature/1  "eng_CaCoolerInlet_Temperature"
  Fcn14/1 -> eng_CaCoolerInlet_pressure/1  "eng_CaCoolerInlet_pressure"
  Bus Selector/7 -> Fcn14/1  "<P2V_mbar>"
  Bus Selector/6 -> Gain2/1  "<AirMassFlow_kgh>"
  Fcn15/1 -> eng_CaCoolerInlet_massfracH2O/1  "eng_CaCoolerInlet_massfracH2O"
  Bus Selector/5 -> Fcn15/1  "<massfracH2O>"
  Gain2/1 -> eng_CaCoolerInlet_mdot/1  "eng_CaCoolerInlet_mdot"
  Fcn12/1 -> eng_T_gas_31/1  "eng_T_gas_31"
  Fcn16/1 -> eng_T_gas_32/1  "eng_T_gas_32"
  Fcn17/1 -> eng_T_gas_2N/1  "eng_T_gas_2N"
  Bus Selector1/1 -> Fcn17/1  "<T2N_degC>"
  Bus Selector1/2 -> Fcn3/1  "<T2S_degC>"
  Bus Selector1/3 -> Fcn4/1  "<P2S_mbar>"
  Bus Selector1/4 -> Fcn5/1  "<AirMassFlow_kgh>"
  Bus Selector1/5 -> Fcn6/1  "<EGRflow_kgh>"
  Bus Selector1/6 -> Fcn12/1  "<T31_degC>"
  Bus Selector1/7 -> Fcn16/1  "<T32_degC>"
  Fcn18/1 -> eng_GasExhaust_molfracCO/1  "eng_GasExhaust_molfracCO"
  Fcn19/1 -> eng_GasExhaust_molfracHC1/1  "eng_GasExhaust_molfracHC1"
  Fcn21/1 -> Add1/1, eng_GasExhaust_molfracNO/1  "eng_GasExhaust_molfracNO"
  Fcn22/1 -> eng_GasExhaust_Temperature/1  "eng_GasExhaust_Temperature"
  Bus Selector2/5 -> Fcn24/1  "<Mfuel_TM1_kgh>"
  Bus Selector2/6 -> Fcn25/1  "<Mfuel_TM1_kg>"
  Bus Selector2/7 -> Fcn26/1  "<Vfuel_TM1_Lh>"
  Bus Selector2/8 -> Fcn23/1  "<Vfuel_TM1_L>"
  Fcn24/1 -> eng_mdot_fuel_TM1/1  "eng_mdot_fuel_TM1"
  Fcn25/1 -> eng_m_fuel_TM1/1  "eng_m_fuel_TM1"
  Fcn26/1 -> eng_vdot_fuel_TM1/1  "eng_vdot_fuel_TM1"
  Fcn23/1 -> eng_v_fuel_TM1/1  "eng_v_fuel_TM1"
  Fcn27/1 -> eng_lambda_exhaust/1  "eng_lambda_exhaust"
  Fcn28/1 -> eng_p_gas_31/1  "eng_p_gas_31"
  Bus Selector1/8 -> Fcn28/1  "<P31_mbar>"
  Bus Selector5/1 -> Fcn29/1  "<T1_degC>"
  Fcn29/1 -> eng_T_gas_1/1  "eng_T_gas_1"
  Fcn30/1 -> eng_T_gas_2/1  "eng_T_gas_2"
  Bus Selector5/2 -> Fcn30/1  "<T2V_degC>"
  Fcn31/1 -> eng_T_gas_6N/1  "eng_T_gas_6N"
  Bus Selector5/3 -> Fcn31/1  "<T6N_degC>"
  Fcn32/1 -> eng_p_gas_2N/1  "eng_p_gas_2N"
  Bus Selector5/4 -> Fcn32/1  "<P2N_mbar>"
  Bus Selector6/1 -> tc_speed_calc_3m/1  "<P2S_mbar>"
  Bus Selector6/2 -> tc_speed_calc_3m/2  "<EngSpeed_rpm>"
  tc_speed_calc_3m/1 -> eng_n_turbocharger/1
  [mcm_wastegate_pos_des] -> eng_wastegate_pos_act/1  "eng_wastegate_pos_act"
  [mcm_egr_valve_pos_des] -> eng_egr_valve_pos_act/1  "eng_egr_valve_pos_act"
  [mcm_am_vcp_pos_des] -> eng_vcp_pos_act/1  "eng_vcp_pos_act"
  [mcm_brkflap_pos_des] -> eng_brkflap_pos_act/1  "eng_brkflap_pos_act"
  Bus Selector7/1 -> Fcn33/1  "<MAdBlue_kgh>"
  Fcn33/1 -> eng_mdot_AdBlue/1  "eng_mdot_AdBlue"
  Fcn34/1 -> eng_vdot_AdBlue/1  "eng_vdot_AdBlue"
  Bus Selector7/2 -> Fcn34/1  "<VAdBlue_Lh>"
  Fcn35/1 -> eng_m_AdBlue/1  "eng_m_AdBlue"
  Bus Selector7/3 -> Fcn35/1  "<MAdBlue_kg>"
  Fcn36/1 -> eng_v_AdBlue/1  "eng_v_AdBlue"
  Bus Selector7/4 -> Fcn36/1  "<VAdBlue_L>"

== system eng_simple_transient_std/eng_simple_transient_std/Pollutant_model ==
  %->ratio : Gain  Gain=-0.01
  Bias : Bias  Bias=1
  Bus Creator4 : BusCreator  Inputs=4
  Constant : Constant  Value=Eng_characteristics_use_mcm_NOx
  Map_CO : Lookup2D  RowIndex=Setpoint_fuelledMode_y_alphaTorque  ColumnIndex=Setpoint_fuelledMode_x_NMOTW_rpm  Table=Setpoint_fuelledMode_z_CO_ppm  LookUpMeth=Interpolation-Use End Values
  Map_HC : Lookup2D  RowIndex=Setpoint_fuelledMode_y_alphaTorque  ColumnIndex=Setpoint_fuelledMode_x_NMOTW_rpm  Table=Setpoint_fuelledMode_z_HC_ppm  LookUpMeth=Interpolation-Use End Values
  Map_NO : Lookup2D  RowIndex=Setpoint_fuelledMode_y_alphaTorque  ColumnIndex=Setpoint_fuelledMode_x_NMOTW_rpm  Table=Setpoint_fuelledMode_z_NO_ppm  LookUpMeth=Interpolation-Use End Values
  Map_NOx : Lookup2D  RowIndex=Setpoint_fuelledMode_y_alphaTorque  ColumnIndex=Setpoint_fuelledMode_x_NMOTW_rpm  Table=Setpoint_fuelledMode_z_NOx_ppm  LookUpMeth=Interpolation-Use End Values
  Product : Product  RndMeth=Zero
  Switch : Switch  Criteria=u2 > Threshold
  Switch1 : Switch  Criteria=u2 > Threshold
  tag scope: Pollutant=global
  wires:
  Bus Creator4/1 -> [Pollutant]  "Pollutant"
  [alphaTorque] -> Map_NO/1, Map_NOx/1, Map_CO/1, Map_HC/1
  [EngSpeed] -> Map_NO/2, Map_NOx/2, Map_CO/2, Map_HC/2
  Map_CO/1 -> Bus Creator4/2  "CO_ppm"
  Map_HC/1 -> Bus Creator4/1  "HC_ppm"
  Map_NOx/1 -> Switch/3  "NOx_ppm"
  Map_NO/1 -> Switch1/3  "NO_ppm"
  Switch1/1 -> Bus Creator4/4  "NO_ppm"
  Switch/1 -> Bus Creator4/3  "NOx_ppm"
  Constant/1 -> Switch/2, Switch1/2
  [mcm_eaf_nox_content_cor] -> Switch/1, Product/1
  [mcm_EngNO2RatioOut_Cval_MCM] -> %->ratio/1
  %->ratio/1 -> Bias/1
  Bias/1 -> Product/2
  Product/1 -> Switch1/1

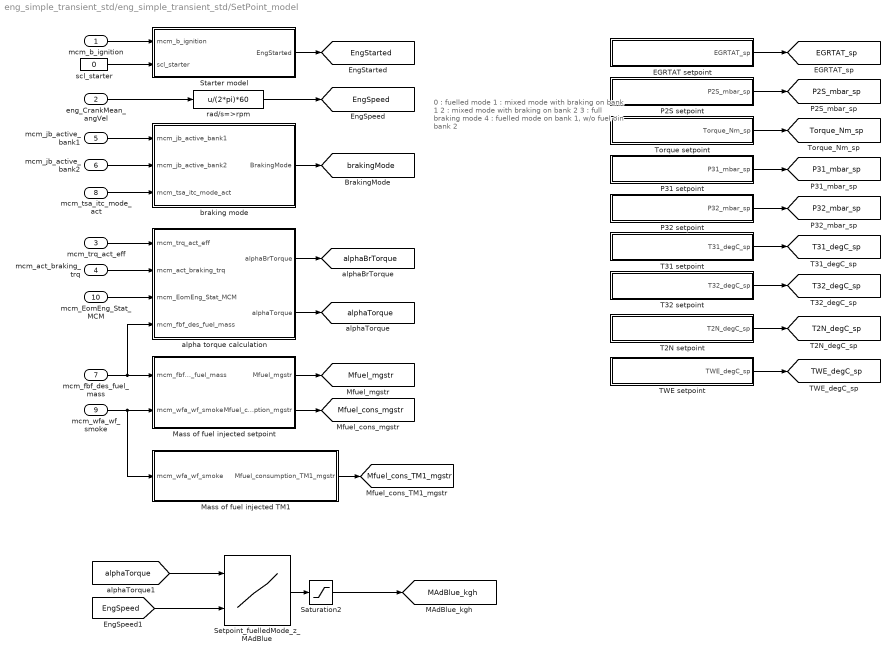
== system eng_simple_transient_std/eng_simple_transient_std/SetPoint_model ==
  note: 0 : fuelled mode
      | 1 : mixed mode with braking on bank 1
      | 2 : mixed mode with braking on bank 2
      | 3 : full braking mode
      | 4 : fuelled mode on bank 1, w/o fuel oin bank 2
  mcm_b_ignition : Inport
  eng_CrankMean_angVel : Inport  Port=2
  mcm_trq_act_eff : Inport  Port=3
  mcm_act_braking_trq : Inport  Port=4
  mcm_jb_active_bank1 : Inport  Port=5
  mcm_jb_active_bank2 : Inport  Port=6
  mcm_fbf_des_fuel_mass : Inport  Port=7
  mcm_tsa_itc_mode_act : Inport  Port=8
  mcm_wfa_wf_smoke : Inport  Port=9
  mcm_EomEng_Stat_MCM : Inport  Port=10
  EGRTAT setpoint : Subsystem
  Mass of fuel injected TM1 : Subsystem
  Mass of fuel injected setpoint : Subsystem
  P2S setpoint : Subsystem
  P31 setpoint : Subsystem
  P32 setpoint : Subsystem
  Saturation2 : Saturate  UpperLimit=1e6  LowerLimit=0
  Setpoint_fuelledMode_z_MAdBlue : Lookup2D  RowIndex=Setpoint_fuelledMode_y_alphaTorque  ColumnIndex=Setpoint_fuelledMode_x_NMOTW_rpm  Table=Setpoint_fuelledMode_z_MAdBlue_kgh
  Starter model : Subsystem
  T2N setpoint : Subsystem
  T31 setpoint : Subsystem
  T32 setpoint : Subsystem
  TWE setpoint : Subsystem
  Torque setpoint : Subsystem
  alpha torque calculation : Subsystem
  braking mode : Subsystem
  rad/s=>rpm : Fcn  Expr=u/(2*pi)*60
  scl_starter : Constant  Value=0
  tag scope: EGRTAT_sp=global, EngSpeed=global, EngStarted=global, MAdBlue_kgh=global, Mfuel_cons_TM1_mgstr=global, Mfuel_cons_mgstr=global, Mfuel_mgstr=global, P2S_mbar_sp=global, P31_mbar_sp=global, P32_mbar_sp=global, T2N_degC_sp=global, T31_degC_sp=global, T32_degC_sp=global, TWE_degC_sp=global, Torque_Nm_sp=global, alphaBrTorque=global, alphaTorque=global, brakingMode=global
  wires:
  rad/s=>rpm/1 -> [EngSpeed]
  scl_starter/1 -> Starter model/2(scl_starter)
  Starter model/1(EngStarted) -> [EngStarted]
  mcm_b_ignition/1 -> Starter model/1(mcm_b_ignition)
  T32 setpoint/1(T32_degC_sp) -> [T32_degC_sp]
  T31 setpoint/1(T31_degC_sp) -> [T31_degC_sp]
  P32 setpoint/1(P32_mbar_sp) -> [P32_mbar_sp]
  P31 setpoint/1(P31_mbar_sp) -> [P31_mbar_sp]
  Torque setpoint/1(Torque_Nm_sp) -> [Torque_Nm_sp]
  P2S setpoint/1(P2S_mbar_sp) -> [P2S_mbar_sp]
  EGRTAT setpoint/1(EGRTAT_sp) -> [EGRTAT_sp]
  Mass of fuel injected setpoint/1(Mfuel_mgstr) -> [Mfuel_mgstr]
  mcm_fbf_des_fuel_mass/1 -> Mass of fuel injected setpoint/1(mcm_fbf_des_fuel_mass), alpha torque calculation/4(mcm_fbf_des_fuel_mass)
  mcm_act_braking_trq/1 -> alpha torque calculation/2(mcm_act_braking_trq)
  mcm_trq_act_eff/1 -> alpha torque calculation/1(mcm_trq_act_eff)
  alpha torque calculation/2(alphaTorque) -> [alphaTorque]
  alpha torque calculation/1(alphaBrTorque) -> [alphaBrTorque]
  braking mode/1(BrakingMode) -> [brakingMode]
  eng_CrankMean_angVel/1 -> rad/s=>rpm/1
  mcm_jb_active_bank2/1 -> braking mode/2(mcm_jb_active_bank2)
  mcm_jb_active_bank1/1 -> braking mode/1(mcm_jb_active_bank1)
  mcm_tsa_itc_mode_act/1 -> braking mode/3(mcm_tsa_itc_mode_act)
  Mass of fuel injected setpoint/2(Mfuel_consumption_mgstr) -> [Mfuel_cons_mgstr]
  mcm_wfa_wf_smoke/1 -> Mass of fuel injected setpoint/2(mcm_wfa_wf_smoke), Mass of fuel injected TM1/1(mcm_wfa_wf_smoke)
  T2N setpoint/1(T2N_degC_sp) -> [T2N_degC_sp]
  Mass of fuel injected TM1/1(Mfuel_consumption_TM1_mgstr) -> [Mfuel_cons_TM1_mgstr]
  Setpoint_fuelledMode_z_MAdBlue/1 -> Saturation2/1
  [EngSpeed] -> Setpoint_fuelledMode_z_MAdBlue/2
  [alphaTorque] -> Setpoint_fuelledMode_z_MAdBlue/1
  Saturation2/1 -> [MAdBlue_kgh]
  TWE setpoint/1(TWE_degC_sp) -> [TWE_degC_sp]
  mcm_EomEng_Stat_MCM/1 -> alpha torque calculation/3(mcm_EomEng_Stat_MCM)

== system eng_simple_transient_std/eng_simple_transient_std/cooler_Input ==
  eng_CoolantEngineOut_Temperature : Inport
  eng_CoolantEngineIn_Temperature : Inport  Port=2
  tag scope: eng_CoolantEngineIn_Temperature=global, eng_CoolantEngineOut_Temperature=global
  wires:
  eng_CoolantEngineOut_Temperature/1 -> [eng_CoolantEngineOut_Temperature]
  eng_CoolantEngineIn_Temperature/1 -> [eng_CoolantEngineIn_Temperature]

== system eng_simple_transient_std/eng_simple_transient_std/Airpath_model/After EGR cooler calculation ==
  Map_EGRcoolerEff : Lookup2D  RowIndex=Airpath_EGRcooler_y_delta_Temp  ColumnIndex=Airpath_EGRcooler_x_EGR_flow  Table=Airpath_EGRcooler_z_efficiency
  T6N : Sum  Inputs=+-
  dT_EGRcooler : Product  Inputs=**
  dT_bfEGRCooler1 : Sum  Inputs=+-
  P6N_mbar : Outport
  T6N_degC : Outport  Port=2
  tag scope: T6N_degC=global
  wires:
  [P2S_mbar] -> P6N_mbar/1
  T6N/1 -> T6N_degC/1, [T6N_degC]
  [EGRflow_kgh] -> Map_EGRcoolerEff/2
  Map_EGRcoolerEff/1 -> dT_EGRcooler/2
  dT_bfEGRCooler1/1 -> dT_EGRcooler/1, Map_EGRcoolerEff/1
  [T6V_degC] -> T6N/1, dT_bfEGRCooler1/1
  dT_EGRcooler/1 -> T6N/2
  [eng_CoolantEngineOut_Temperature] -> dT_bfEGRCooler1/2

== system eng_simple_transient_std/eng_simple_transient_std/Airpath_model/After air cooler calculation ==
  Map_AirCoolerEff : Lookup2D  RowIndex=Airpath_aircooler_y_delta_Temp  ColumnIndex=Airpath_aircooler_x_ML_kgh  Table=Airpath_aircooler_z_efficiency  LookUpMeth=Interpolation-Use End Values
  T2N Flow : Sum  Inputs=+-
  T2N sensor filter : Subsystem  AncestorBlock=ControlLib/# First order filter
  dT_AirCooler : Product  Inputs=**
  dT_bfAirCooler : Sum  Inputs=+-
  P2N_mbar : Outport
  T2N_degC : Outport  Port=2
  tag scope: T2N_degC_wf=global
  wires:
  [P2S_mbar] -> P2N_mbar/1
  T2N sensor filter/1(T2N_degC) -> T2N_degC/1
  dT_AirCooler/1 -> T2N Flow/2
  [AirMassFlow_kgh] -> Map_AirCoolerEff/2
  [T2V_degC] -> T2N Flow/1, dT_bfAirCooler/1
  T2N Flow/1 -> [T2N_degC_wf], T2N sensor filter/1(T2N_flow_degC)
  dT_bfAirCooler/1 -> Map_AirCoolerEff/1, dT_AirCooler/1
  Map_AirCoolerEff/1 -> dT_AirCooler/2
  [env_AirTemp] -> dT_bfAirCooler/2

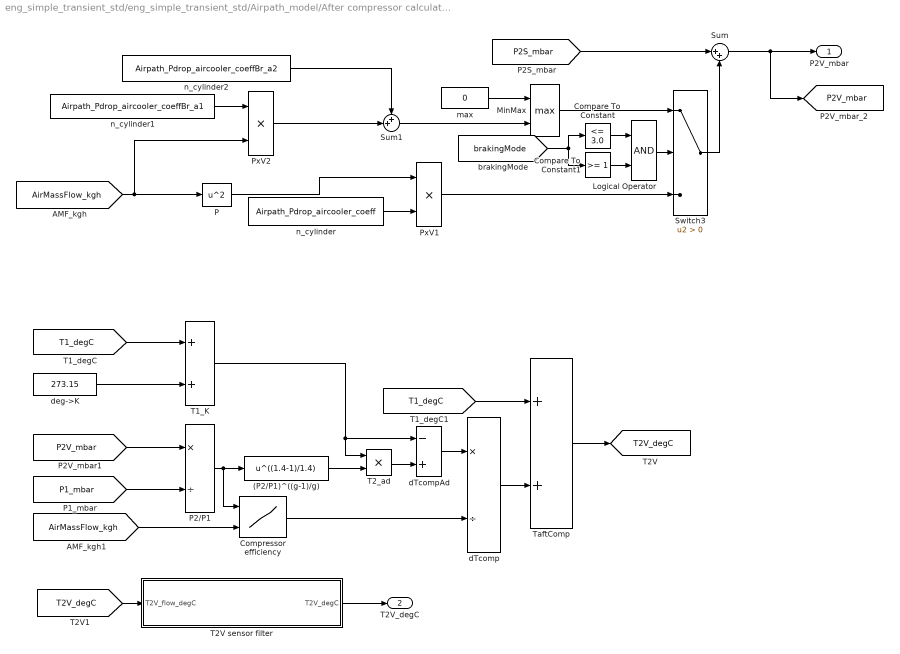
== system eng_simple_transient_std/eng_simple_transient_std/Airpath_model/After compressor calculation ==
  (P2/P1)^((g-1)/g) : Fcn  Expr=u^((1.4-1)/1.4)
  Compare To Constant : simulink/Logic and Bit Operations/Compare To Constant  relop=<=  const=3.0  OutDataTypeStr=uint8
  Compare To Constant1 : simulink/Logic and Bit Operations/Compare To Constant  relop=>=  const=1  OutDataTypeStr=uint8
  Compressor efficiency : Lookup2D  RowIndex=Airpath_compressor_y_PressRatio  ColumnIndex=Airpath_compressor_x_massFlow_kgh  Table=Airpath_compressor_z_Efficiency  LookUpMeth=Interpolation-Use End Values
  Logical Operator : Logic  AllPortsSameDT=off  OutDataTypeStr=boolean
  MinMax : MinMax  Function=max  Inputs=2
  P : Fcn  Expr=u^2
  P2/P1 : Product  Inputs=*/
  PxV1 : Product  RndMeth=Zero
  PxV2 : Product  RndMeth=Zero
  Sum : Sum  Inputs=|++
  Sum1 : Sum  Inputs=++|
  Switch3 : Switch  Criteria=u2 > Threshold
  T1_K : Sum
  T2V sensor filter : Subsystem  AncestorBlock=ControlLib/# First order filter
  T2_ad : Product  Inputs=**
  TaftComp : Sum
  dTcomp : Product  Inputs=*/
  dTcompAd : Sum  Inputs=-+
  deg->K : Constant  Value=273.15
  max : Constant  Value=0
  n_cylinder : Constant  Value=Airpath_Pdrop_aircooler_coeff
  n_cylinder1 : Constant  Value=Airpath_Pdrop_aircooler_coeffBr_a1
  n_cylinder2 : Constant  Value=Airpath_Pdrop_aircooler_coeffBr_a2
  P2V_mbar : Outport
  T2V_degC : Outport  Port=2
  tag scope: P2V_mbar=global, T2V_degC=global
  wires:
  PxV2/1 -> Sum1/2
  n_cylinder2/1 -> Sum1/1
  n_cylinder1/1 -> PxV2/1
  PxV1/1 -> Switch3/3
  n_cylinder/1 -> PxV1/2
  P/1 -> PxV1/1
  [T1_degC] -> TaftComp/1
  [T2V_degC] -> T2V sensor filter/1(T2V_flow_degC)
  P2/P1/1 -> (P2/P1)^((g-1)/g)/1, Compressor efficiency/1
  [P1_mbar] -> P2/P1/2
  [T1_degC] -> T1_K/1
  (P2/P1)^((g-1)/g)/1 -> T2_ad/2
  deg->K/1 -> T1_K/2
  T1_K/1 -> dTcompAd/1, T2_ad/1
  T2_ad/1 -> dTcompAd/2
  dTcompAd/1 -> dTcomp/1
  Compressor efficiency/1 -> dTcomp/2
  TaftComp/1 -> [T2V_degC]
  dTcomp/1 -> TaftComp/2
  [P2V_mbar] -> P2/P1/1
  [AirMassFlow_kgh] -> Compressor efficiency/2
  T2V sensor filter/1(T2V_degC) -> T2V_degC/1
  Sum1/1 -> MinMax/2
  Switch3/1 -> Sum/2
  MinMax/1 -> Switch3/1
  max/1 -> MinMax/1
  Sum/1 -> [P2V_mbar], P2V_mbar/1
  [P2S_mbar] -> Sum/1
  [AirMassFlow_kgh] -> PxV2/2, P/1
  [brakingMode] -> Compare To Constant/1, Compare To Constant1/1
  Compare To Constant/1 -> Logical Operator/1
  Compare To Constant1/1 -> Logical Operator/2
  Logical Operator/1 -> Switch3/2

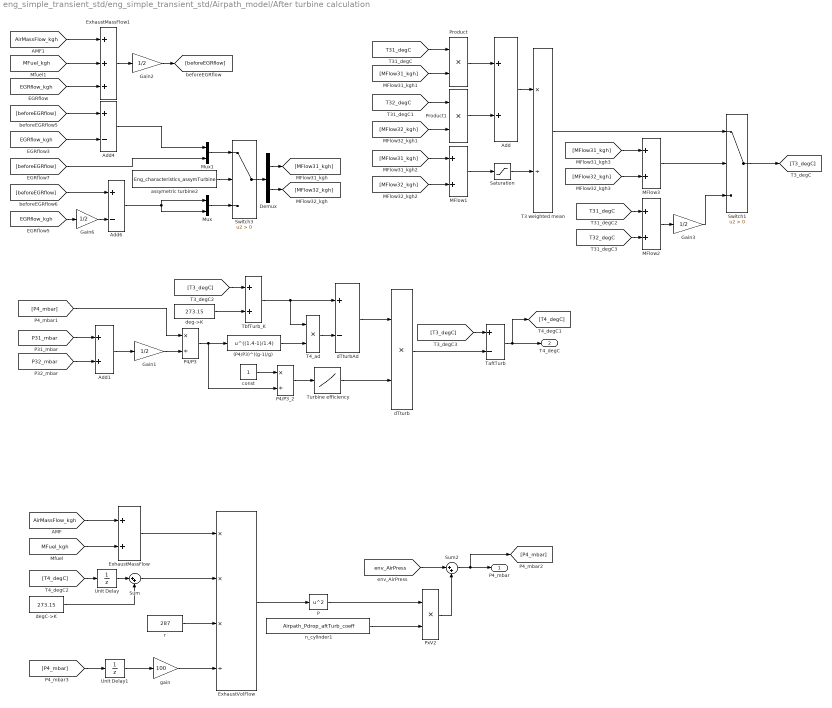
== system eng_simple_transient_std/eng_simple_transient_std/Airpath_model/After turbine calculation ==
  (P4/P3)^((g-1)/g) : Fcn  Expr=u^((1.4-1)/1.4)
  Add : Sum
  Add1 : Sum
  Add4 : Sum  Inputs=+-
  Add6 : Sum  Inputs=+-
  Demux : Demux  Outputs=2
  ExhaustMassFlow : Sum
  ExhaustMassFlow1 : Sum  Inputs=+++
  ExhaustVolFlow : Product  Inputs=***/
  Gain{1..3,6} (4 alike) : Gain  Gain=1/2
  MFlow1 : Sum
  MFlow2 : Sum
  MFlow3 : Sum
  Mux : Mux  Inputs=2
  Mux1 : Mux  Inputs=2
  P : Fcn  Expr=u^2
  P4/P3 : Product  Inputs=*/
  P4/P3_2 : Product  Inputs=*/
  Product : Product  RndMeth=Zero
  Product1 : Product  RndMeth=Zero
  PxV2 : Product  RndMeth=Zero
  Saturation : Saturate  UpperLimit=inf  LowerLimit=0.1
  Sum : Sum  Inputs=|++
  Sum2 : Sum  Inputs=|++
  Switch1 : Switch  Criteria=u2 > Threshold
  Switch3 : Switch  Criteria=u2 > Threshold
  T3 weighted mean : Product  Inputs=*/
  T4_ad : Product  Inputs=**
  TaftTurb : Sum  Inputs=+-
  TbfTurb_K : Sum
  Turbine efficiency : Lookup  InputValues=Airpath_turbine_x_PressRatio  Table=Airpath_turbine_y_Efficiency
  Unit Delay : UnitDelay  InitialCondition=20  SampleTime=-1
  Unit Delay1 : UnitDelay  InitialCondition=1000  SampleTime=-1
  assymetric turbine2 : Constant  Value=Eng_characteristics_assymTurbine
  const : Constant
  dTturb : Product  Inputs=**
  dTturbAd : Sum  Inputs=+-
  deg->K : Constant  Value=273.15
  degC->K : Constant  Value=273.15
  gain : Gain  Gain=100
  n_cylinder1 : Constant  Value=Airpath_Pdrop_aftTurb_coeff
  r : Constant  Value=287
  P4_mbar : Outport
  T4_degC : Outport  Port=2
  wires:
  P/1 -> PxV2/1
  n_cylinder1/1 -> PxV2/2
  MFlow3/1 -> Switch1/2
  [MFlow32_kgh] -> MFlow3/2
  [MFlow31_kgh] -> MFlow3/1
  Saturation/1 -> T3 weighted mean/2
  Gain3/1 -> Switch1/3
  MFlow2/1 -> Gain3/1
  [T32_degC] -> MFlow2/2
  [T31_degC] -> MFlow2/1
  T3 weighted mean/1 -> Switch1/1
  Switch1/1 -> [T3_degC]
  Demux/2 -> [MFlow32_kgh]
  Switch3/1 -> Demux/1
  Demux/1 -> [MFlow31_kgh]
  Add4/1 -> Mux1/1
  Mux1/1 -> Switch3/1
  Add6/1 -> Mux/2, Mux/1
  Mux/1 -> Switch3/3
  assymetric turbine2/1 -> Switch3/2
  Gain6/1 -> Add6/2
  [EGRflow_kgh] -> Gain6/1
  [beforeEGRflow] -> Add6/1
  [EGRflow_kgh] -> Add4/2
  [beforeEGRflow] -> Add4/1
  Gain2/1 -> [beforeEGRflow]
  [EGRflow_kgh] -> ExhaustMassFlow1/3
  Add/1 -> T3 weighted mean/1
  MFlow1/1 -> Saturation/1
  [MFlow32_kgh] -> MFlow1/2
  [MFlow31_kgh] -> MFlow1/1
  Product1/1 -> Add/2
  Product/1 -> Add/1
  [MFlow32_kgh] -> Product1/2
  [T32_degC] -> Product1/1
  [MFlow31_kgh] -> Product/2
  [T31_degC] -> Product/1
  ExhaustMassFlow1/1 -> Gain2/1
  [AirMassFlow_kgh] -> ExhaustMassFlow1/1
  [MFuel_kgh] -> ExhaustMassFlow1/2
  [P4_mbar] -> Unit Delay1/1
  gain/1 -> ExhaustVolFlow/4
  PxV2/1 -> Sum2/2
  ExhaustVolFlow/1 -> P/1
  Unit Delay1/1 -> gain/1
  r/1 -> ExhaustVolFlow/3
  Sum/1 -> ExhaustVolFlow/2
  Unit Delay/1 -> Sum/1
  degC->K/1 -> Sum/2
  [T4_degC] -> Unit Delay/1
  [AirMassFlow_kgh] -> ExhaustMassFlow/1
  [env_AirPress] -> Sum2/1
  Sum2/1 -> [P4_mbar], P4_mbar/1
  ExhaustMassFlow/1 -> ExhaustVolFlow/1
  [MFuel_kgh] -> ExhaustMassFlow/2
  [T3_degC] -> TaftTurb/1
  [P32_mbar] -> Add1/2
  [P31_mbar] -> Add1/1
  [T3_degC] -> TbfTurb_K/1
  const/1 -> P4/P3_2/1
  P4/P3_2/1 -> Turbine efficiency/1
  [P4_mbar] -> P4/P3/1
  Gain1/1 -> P4/P3/2
  Add1/1 -> Gain1/1
  P4/P3/1 -> (P4/P3)^((g-1)/g)/1, P4/P3_2/2
  (P4/P3)^((g-1)/g)/1 -> T4_ad/2
  deg->K/1 -> TbfTurb_K/2
  TbfTurb_K/1 -> dTturbAd/1, T4_ad/1
  T4_ad/1 -> dTturbAd/2
  dTturbAd/1 -> dTturb/1
  Turbine efficiency/1 -> dTturb/2
  TaftTurb/1 -> [T4_degC], T4_degC/1
  dTturb/1 -> TaftTurb/2
  [beforeEGRflow] -> Mux1/2

== system eng_simple_transient_std/eng_simple_transient_std/Airpath_model/Airbox calculation ==
  FT_AIR : Product  RndMeth=Zero
  FT_AIR+FT_EGR : Sum
  FT_EGR : Product  RndMeth=Zero
  Intake_flow_kgh : Sum
  P2S filter : Subsystem  AncestorBlock=ControlLib/# First order filter
  PxV2 : Product  RndMeth=Zero
  Saturation : Saturate  UpperLimit=inf  LowerLimit=0.1
  Saturation1 : Saturate  UpperLimit=inf  LowerLimit=0
  Saturation2 : Saturate  UpperLimit=inf  LowerLimit=0.1
  Switch1 : Switch  Criteria=u2 > Threshold
  T2S sensor filter : Subsystem  AncestorBlock=ControlLib/# First order filter
  Tairbox : Product  Inputs=*/
  n_cylinder1 : Constant  Value=Airpath_Tairbox_EGR_coeff
  P2S_mbar : Outport
  T2S_degC : Outport  Port=2
  tag scope: P2S_mbar=global, T2S_degC=global
  wires:
  [T6N_degC] -> FT_EGR/1
  n_cylinder1/1 -> PxV2/2
  [env_AirTemp] -> Switch1/3
  Tairbox/1 -> Switch1/1
  Switch1/1 -> T2S sensor filter/1(T2S_flow_degC)
  [EngStarted] -> Switch1/2
  T2S sensor filter/1(T2S_degC) -> [T2S_degC], T2S_degC/1
  PxV2/1 -> FT_EGR/2, Intake_flow_kgh/2
  [EGRflow_kgh] -> Saturation1/1
  [AirMassFlow_kgh] -> Saturation/1
  [AirMassFlow_kgh] -> Saturation2/1
  [T2N_degC_wf] -> FT_AIR/1
  FT_AIR+FT_EGR/1 -> Tairbox/1
  FT_AIR/1 -> FT_AIR+FT_EGR/1
  FT_EGR/1 -> FT_AIR+FT_EGR/2
  Intake_flow_kgh/1 -> Tairbox/2
  P2S filter/1(P2S_mbar) -> [P2S_mbar], P2S_mbar/1
  [P2S_mbar_sp] -> P2S filter/1(P2S_mbar_sp)
  Saturation1/1 -> PxV2/1
  Saturation/1 -> Intake_flow_kgh/1
  Saturation2/1 -> FT_AIR/2

== system eng_simple_transient_std/eng_simple_transient_std/Airpath_model/Before EGR cooler calculation ==
  P6V_mbar : Outport
  T6V_degC : Outport  Port=2
  tag scope: T6V_degC=global
  wires:
  [P31_mbar] -> P6V_mbar/1
  [T31_degC] -> [T6V_degC], T6V_degC/1

== system eng_simple_transient_std/eng_simple_transient_std/Airpath_model/Before compressor calculation ==
  Pdrop_bfrComp : Product  RndMeth=Zero
  Sum : Sum  Inputs=|+-
  a : Fcn  Expr=u^2
  n_cylinder : Constant  Value=Airpath_Pdrop_bfrComp_coeff
  massfracH2O : Outport
  P1_mbar : Outport  Port=2
  T1_degC : Outport  Port=3
  tag scope: P1_mbar=global, T1_degC=global
  wires:
  Pdrop_bfrComp/1 -> Sum/2
  n_cylinder/1 -> Pdrop_bfrComp/2
  a/1 -> Pdrop_bfrComp/1
  [AirMassFlow_kgh] -> a/1
  [env_AirH2OMassFrac] -> massfracH2O/1
  [env_AirPress] -> Sum/1
  [env_AirTemp] -> [T1_degC], T1_degC/1
  Sum/1 -> [P1_mbar], P1_mbar/1

== system eng_simple_transient_std/eng_simple_transient_std/Airpath_model/Before turbine calculation ==
  P31 filter : Subsystem  AncestorBlock=ControlLib/# First order filter
  P32 filter : Subsystem  AncestorBlock=ControlLib/# First order filter
  T31 filter : Subsystem  AncestorBlock=ControlLib/# First order filter
  T32 filter : Subsystem  AncestorBlock=ControlLib/# First order filter
  P31_mbar : Outport
  T31_degC : Outport  Port=2
  P32_mbar : Outport  Port=3
  T32_degC : Outport  Port=4
  tag scope: P31_mbar=global, P32_mbar=global, T31_degC=global, T32_degC=global
  wires:
  T32 filter/1(T32_degC) -> [T32_degC], T32_degC/1
  [T32_degC_sp] -> T32 filter/1(T32_degC_sp)
  [P32_mbar_sp] -> P32 filter/1(P32_mbar_sp)
  P32 filter/1(P32_mbar) -> [P32_mbar], P32_mbar/1
  T31 filter/1(T31_degC) -> [T31_degC], T31_degC/1
  [T31_degC_sp] -> T31 filter/1(T31_degC_sp)
  [P31_mbar_sp] -> P31 filter/1(P31_mbar_sp)
  P31 filter/1(P31_mbar) -> [P31_mbar], P31_mbar/1
